simulink model "TST_EnvP_DD"  (R2016b)
settings: Solver=FixedStepDiscrete  StartTime=0.0  StopTime=simTime  FixedStep=sampleTime  RelTol=1e-3
values from neighbouring files (symbols this model uses):
  testCase = 1    [initTST_EnvP_DD_001.m]    (also in initTST_EnvP_DD_002.m = 2; initTST_EnvP_DD_003.m = 3; initTST_EnvP_DD_004.m = 4)
libraries: simulink x41, UnitTest_Lib x36
settings Model: Creator=liangyunbo  LastModifiedBy=liangyunbo
settings DebuggingCC: SignalRangeChecking=error

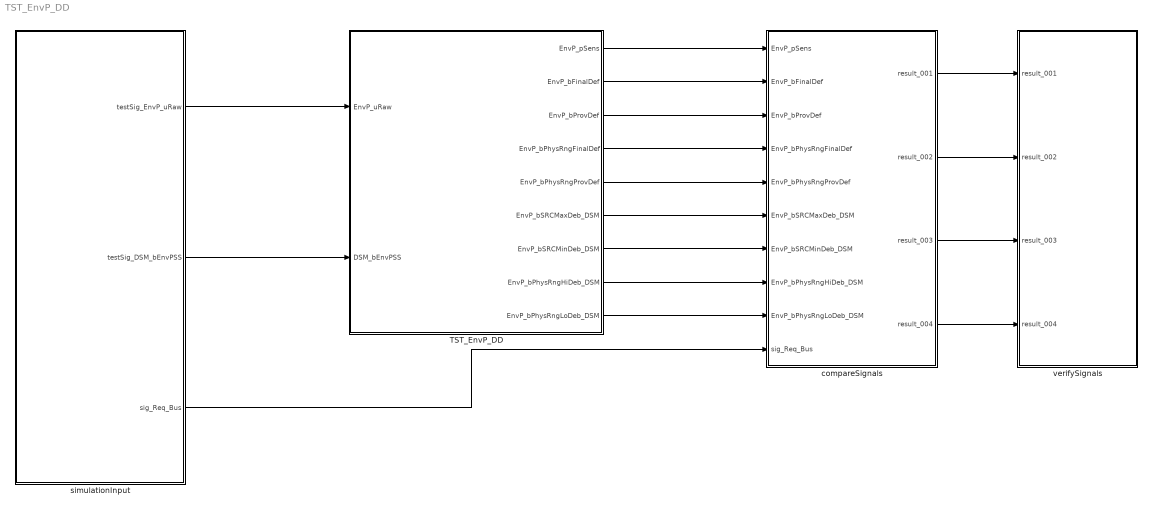
== system TST_EnvP_DD ==
  TST_EnvP_DD : Subsystem
  compareSignals : Subsystem
  simulationInput : Subsystem
  verifySignals : Subsystem
  wires:
  simulationInput/1(testSig_EnvP_uRaw) -> TST_EnvP_DD/1(EnvP_uRaw)
  simulationInput/2(testSig_DSM_bEnvPSS) -> TST_EnvP_DD/2(DSM_bEnvPSS)
  TST_EnvP_DD/1(EnvP_pSens) -> compareSignals/1(EnvP_pSens)
  TST_EnvP_DD/2(EnvP_bFinalDef) -> compareSignals/2(EnvP_bFinalDef)
  TST_EnvP_DD/3(EnvP_bProvDef) -> compareSignals/3(EnvP_bProvDef)
  TST_EnvP_DD/4(EnvP_bPhysRngFinalDef) -> compareSignals/4(EnvP_bPhysRngFinalDef)
  TST_EnvP_DD/5(EnvP_bPhysRngProvDef) -> compareSignals/5(EnvP_bPhysRngProvDef)
  TST_EnvP_DD/6(EnvP_bSRCMaxDeb_DSM) -> compareSignals/6(EnvP_bSRCMaxDeb_DSM)
  TST_EnvP_DD/7(EnvP_bSRCMinDeb_DSM) -> compareSignals/7(EnvP_bSRCMinDeb_DSM)
  TST_EnvP_DD/8(EnvP_bPhysRngHiDeb_DSM) -> compareSignals/8(EnvP_bPhysRngHiDeb_DSM)
  TST_EnvP_DD/9(EnvP_bPhysRngLoDeb_DSM) -> compareSignals/9(EnvP_bPhysRngLoDeb_DSM)
  simulationInput/3(sig_Req_Bus) -> compareSignals/10(sig_Req_Bus)
  compareSignals/1(result_001) -> verifySignals/1(result_001)
  compareSignals/2(result_002) -> verifySignals/2(result_002)
  compareSignals/3(result_003) -> verifySignals/3(result_003)
  compareSignals/4(result_004) -> verifySignals/4(result_004)

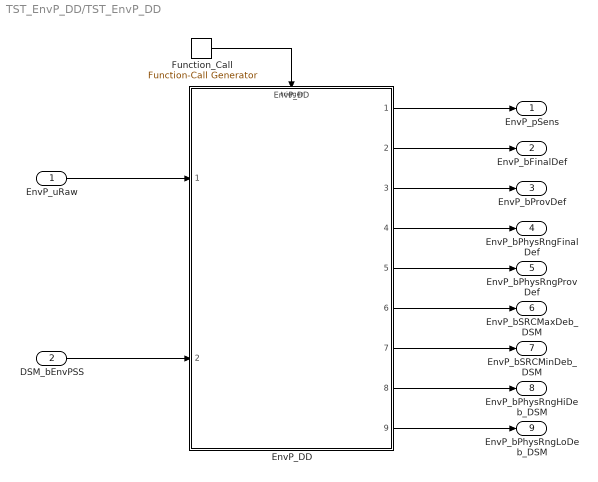
== system TST_EnvP_DD/TST_EnvP_DD ==
  EnvP_uRaw : Inport
  DSM_bEnvPSS : Inport  Port=2
  EnvP_DD : ModelReference  ModelNameDialog=EnvP_DD  SimulationMode=Normal  ModelReferenceVersion=1.9  TriggerPortName=function  TriggerPortTriggerType=function-call  TriggerPortStatesWhenEnabling=held
  Function_Call : simulink/Ports & Subsystems/Function-Call Generator  sample_time=sampleTime  numberOfIterations=1
  EnvP_pSens : Outport
  EnvP_bFinalDef : Outport  Port=2
  EnvP_bProvDef : Outport  Port=3
  EnvP_bPhysRngFinalDef : Outport  Port=4
  EnvP_bPhysRngProvDef : Outport  Port=5
  EnvP_bSRCMaxDeb_DSM : Outport  Port=6
  EnvP_bSRCMinDeb_DSM : Outport  Port=7
  EnvP_bPhysRngHiDeb_DSM : Outport  Port=8
  EnvP_bPhysRngLoDeb_DSM : Outport  Port=9
  wires:
  Function_Call/1 -> EnvP_DD/Trigger
  EnvP_uRaw/1 -> EnvP_DD/1
  DSM_bEnvPSS/1 -> EnvP_DD/2
  EnvP_DD/1 -> EnvP_pSens/1
  EnvP_DD/2 -> EnvP_bFinalDef/1
  EnvP_DD/3 -> EnvP_bProvDef/1
  EnvP_DD/4 -> EnvP_bPhysRngFinalDef/1
  EnvP_DD/5 -> EnvP_bPhysRngProvDef/1
  EnvP_DD/6 -> EnvP_bSRCMaxDeb_DSM/1
  EnvP_DD/7 -> EnvP_bSRCMinDeb_DSM/1
  EnvP_DD/8 -> EnvP_bPhysRngHiDeb_DSM/1
  EnvP_DD/9 -> EnvP_bPhysRngLoDeb_DSM/1

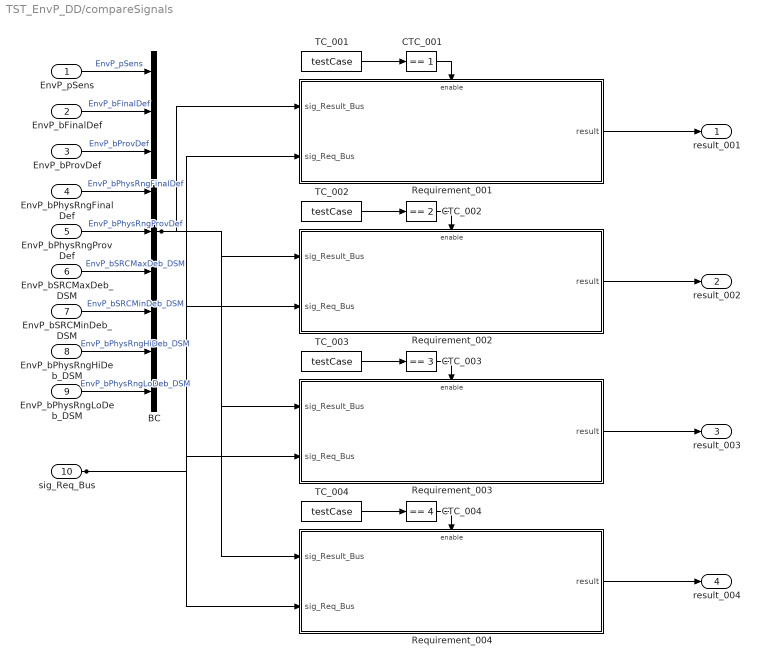
== system TST_EnvP_DD/compareSignals ==
  EnvP_pSens : Inport
  EnvP_bFinalDef : Inport  Port=2
  EnvP_bProvDef : Inport  Port=3
  EnvP_bPhysRngFinalDef : Inport  Port=4
  EnvP_bPhysRngProvDef : Inport  Port=5
  EnvP_bSRCMaxDeb_DSM : Inport  Port=6
  EnvP_bSRCMinDeb_DSM : Inport  Port=7
  EnvP_bPhysRngHiDeb_DSM : Inport  Port=8
  EnvP_bPhysRngLoDeb_DSM : Inport  Port=9
  sig_Req_Bus : Inport  Port=10
  BC : BusCreator  Inputs=9
  CTC_001 : simulink/Logic and Bit Operations/Compare To Constant  relop===  const=1  OutDataTypeStr=boolean
  CTC_002 : simulink/Logic and Bit Operations/Compare To Constant  relop===  const=2  OutDataTypeStr=boolean
  CTC_003 : simulink/Logic and Bit Operations/Compare To Constant  relop===  const=3  OutDataTypeStr=boolean
  CTC_004 : simulink/Logic and Bit Operations/Compare To Constant  relop===  const=4  OutDataTypeStr=boolean
  Requirement_001 : Subsystem
  Requirement_002 : Subsystem
  Requirement_003 : Subsystem
  Requirement_004 : Subsystem
  TC_001 : Constant  Value=testCase
  TC_002 : Constant  Value=testCase
  TC_003 : Constant  Value=testCase
  TC_004 : Constant  Value=testCase
  result_001 : Outport
  result_002 : Outport  Port=2
  result_003 : Outport  Port=3
  result_004 : Outport  Port=4
  wires:
  EnvP_pSens/1 -> BC/1  "EnvP_pSens"
  EnvP_bFinalDef/1 -> BC/2  "EnvP_bFinalDef"
  EnvP_bProvDef/1 -> BC/3  "EnvP_bProvDef"
  EnvP_bPhysRngFinalDef/1 -> BC/4  "EnvP_bPhysRngFinalDef"
  EnvP_bPhysRngProvDef/1 -> BC/5  "EnvP_bPhysRngProvDef"
  EnvP_bSRCMaxDeb_DSM/1 -> BC/6  "EnvP_bSRCMaxDeb_DSM"
  EnvP_bSRCMinDeb_DSM/1 -> BC/7  "EnvP_bSRCMinDeb_DSM"
  EnvP_bPhysRngHiDeb_DSM/1 -> BC/8  "EnvP_bPhysRngHiDeb_DSM"
  EnvP_bPhysRngLoDeb_DSM/1 -> BC/9  "EnvP_bPhysRngLoDeb_DSM"
  TC_001/1 -> CTC_001/1
  CTC_001/1 -> Requirement_001/Enable
  sig_Req_Bus/1 -> Requirement_001/2(sig_Req_Bus), Requirement_002/2(sig_Req_Bus), Requirement_003/2(sig_Req_Bus), Requirement_004/2(sig_Req_Bus)
  BC/1 -> Requirement_001/1(sig_Result_Bus), Requirement_002/1(sig_Result_Bus), Requirement_003/1(sig_Result_Bus), Requirement_004/1(sig_Result_Bus)
  Requirement_001/1(result) -> result_001/1
  TC_002/1 -> CTC_002/1
  CTC_002/1 -> Requirement_002/Enable
  Requirement_002/1(result) -> result_002/1
  TC_003/1 -> CTC_003/1
  CTC_003/1 -> Requirement_003/Enable
  Requirement_003/1(result) -> result_003/1
  TC_004/1 -> CTC_004/1
  CTC_004/1 -> Requirement_004/Enable
  Requirement_004/1(result) -> result_004/1

== system TST_EnvP_DD/simulationInput ==
  BS : BusSelector  OutputSignals=testSig_EnvP_uRaw,testSig_DSM_bEnvPSS
  MPSw : MultiPortSwitch  Inputs=4  SaturateOnIntegerOverflow=on  InputSameDT=on
  TestCase : Constant  Value=testCase
  testSignals_R001 : Subsystem
  testSignals_R002 : Subsystem
  testSignals_R003 : Subsystem
  testSignals_R004 : Subsystem
  testSig_EnvP_uRaw : Outport
  testSig_DSM_bEnvPSS : Outport  Port=2
  sig_Req_Bus : Outport  Port=3
  wires:
  BS/1 -> testSig_EnvP_uRaw/1  "<testSig_EnvP_uRaw>"
  BS/2 -> testSig_DSM_bEnvPSS/1  "<testSig_DSM_bEnvPSS>"
  MPSw/1 -> BS/1, sig_Req_Bus/1
  TestCase/1 -> MPSw/1
  testSignals_R001/1(testSignals) -> MPSw/2
  testSignals_R002/1(testSignals) -> MPSw/3
  testSignals_R003/1(testSignals) -> MPSw/4
  testSignals_R004/1(testSignals) -> MPSw/5

== system TST_EnvP_DD/verifySignals ==
  result_001 : Inport
  result_002 : Inport  Port=2
  result_003 : Inport  Port=3
  result_004 : Inport  Port=4
  Assertion_001 : Assertion  Enabled=off
  Assertion_002 : Assertion  Enabled=off
  Assertion_003 : Assertion  Enabled=off
  Assertion_004 : Assertion  Enabled=off
  wires:
  result_001/1 -> Assertion_001/1
  result_002/1 -> Assertion_002/1
  result_003/1 -> Assertion_003/1
  result_004/1 -> Assertion_004/1

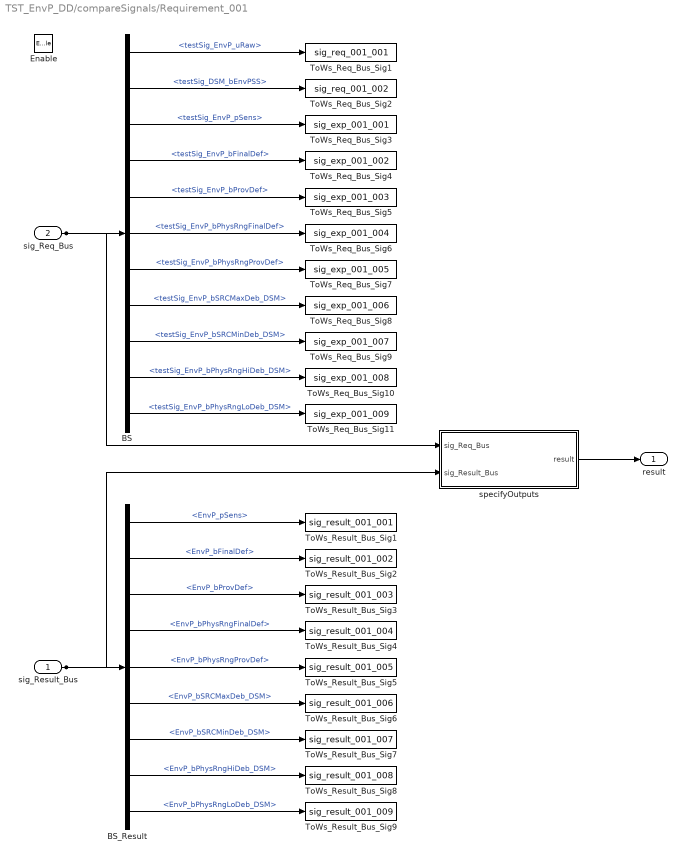
== system TST_EnvP_DD/compareSignals/Requirement_001 ==
  sig_Result_Bus : Inport
  sig_Req_Bus : Inport  Port=2
  Enable : EnablePort
  BS : BusSelector  OutputSignals=testSig_EnvP_uRaw,testSig_DSM_bEnvPSS,testSig_EnvP_pSens,testSig_EnvP_bFinalDef,testSig_EnvP_bProvDef,testSig_EnvP_bPhysRngFinalDef,testSig_EnvP_bPhysRngProvDef,testSig_EnvP_bSRCMaxDeb_DSM,testSig_EnvP_bSRCMinDeb_DSM,testSig_EnvP_bPhysRngHiDeb_DSM,testSig_EnvP_bPhysRngLoDeb_DSM
  BS_Result : BusSelector  OutputSignals=EnvP_pSens,EnvP_bFinalDef,EnvP_bProvDef,EnvP_bPhysRngFinalDef,EnvP_bPhysRngProvDef,EnvP_bSRCMaxDeb_DSM,EnvP_bSRCMinDeb_DSM,EnvP_bPhysRngHiDeb_DSM,EnvP_bPhysRngLoDeb_DSM
  ToWs_Req_Bus_Sig1 : ToWorkspace  VariableName=sig_req_001_001  SaveFormat=Structure With Time
  ToWs_Req_Bus_Sig10 : ToWorkspace  VariableName=sig_exp_001_008  SaveFormat=Structure With Time
  ToWs_Req_Bus_Sig11 : ToWorkspace  VariableName=sig_exp_001_009  SaveFormat=Structure With Time
  ToWs_Req_Bus_Sig2 : ToWorkspace  VariableName=sig_req_001_002  SaveFormat=Structure With Time
  ToWs_Req_Bus_Sig3 : ToWorkspace  VariableName=sig_exp_001_001  SaveFormat=Structure With Time
  ToWs_Req_Bus_Sig4 : ToWorkspace  VariableName=sig_exp_001_002  SaveFormat=Structure With Time
  ToWs_Req_Bus_Sig5 : ToWorkspace  VariableName=sig_exp_001_003  SaveFormat=Structure With Time
  ToWs_Req_Bus_Sig6 : ToWorkspace  VariableName=sig_exp_001_004  SaveFormat=Structure With Time
  ToWs_Req_Bus_Sig7 : ToWorkspace  VariableName=sig_exp_001_005  SaveFormat=Structure With Time
  ToWs_Req_Bus_Sig8 : ToWorkspace  VariableName=sig_exp_001_006  SaveFormat=Structure With Time
  ToWs_Req_Bus_Sig9 : ToWorkspace  VariableName=sig_exp_001_007  SaveFormat=Structure With Time
  ToWs_Result_Bus_Sig1 : ToWorkspace  VariableName=sig_result_001_001  SaveFormat=Structure With Time
  ToWs_Result_Bus_Sig2 : ToWorkspace  VariableName=sig_result_001_002  SaveFormat=Structure With Time
  ToWs_Result_Bus_Sig3 : ToWorkspace  VariableName=sig_result_001_003  SaveFormat=Structure With Time
  ToWs_Result_Bus_Sig4 : ToWorkspace  VariableName=sig_result_001_004  SaveFormat=Structure With Time
  ToWs_Result_Bus_Sig5 : ToWorkspace  VariableName=sig_result_001_005  SaveFormat=Structure With Time
  ToWs_Result_Bus_Sig6 : ToWorkspace  VariableName=sig_result_001_006  SaveFormat=Structure With Time
  ToWs_Result_Bus_Sig7 : ToWorkspace  VariableName=sig_result_001_007  SaveFormat=Structure With Time
  ToWs_Result_Bus_Sig8 : ToWorkspace  VariableName=sig_result_001_008  SaveFormat=Structure With Time
  ToWs_Result_Bus_Sig9 : ToWorkspace  VariableName=sig_result_001_009  SaveFormat=Structure With Time
  specifyOutputs : Subsystem
  result : Outport
  wires:
  sig_Req_Bus/1 -> BS/1, specifyOutputs/1(sig_Req_Bus)
  BS/1 -> ToWs_Req_Bus_Sig1/1  "<testSig_EnvP_uRaw>"
  BS/2 -> ToWs_Req_Bus_Sig2/1  "<testSig_DSM_bEnvPSS>"
  BS/3 -> ToWs_Req_Bus_Sig3/1  "<testSig_EnvP_pSens>"
  BS/4 -> ToWs_Req_Bus_Sig4/1  "<testSig_EnvP_bFinalDef>"
  BS/5 -> ToWs_Req_Bus_Sig5/1  "<testSig_EnvP_bProvDef>"
  BS/6 -> ToWs_Req_Bus_Sig6/1  "<testSig_EnvP_bPhysRngFinalDef>"
  BS/7 -> ToWs_Req_Bus_Sig7/1  "<testSig_EnvP_bPhysRngProvDef>"
  BS/8 -> ToWs_Req_Bus_Sig8/1  "<testSig_EnvP_bSRCMaxDeb_DSM>"
  BS/9 -> ToWs_Req_Bus_Sig9/1  "<testSig_EnvP_bSRCMinDeb_DSM>"
  BS/10 -> ToWs_Req_Bus_Sig10/1  "<testSig_EnvP_bPhysRngHiDeb_DSM>"
  BS/11 -> ToWs_Req_Bus_Sig11/1  "<testSig_EnvP_bPhysRngLoDeb_DSM>"
  sig_Result_Bus/1 -> BS_Result/1, specifyOutputs/2(sig_Result_Bus)
  BS_Result/1 -> ToWs_Result_Bus_Sig1/1  "<EnvP_pSens>"
  BS_Result/2 -> ToWs_Result_Bus_Sig2/1  "<EnvP_bFinalDef>"
  BS_Result/3 -> ToWs_Result_Bus_Sig3/1  "<EnvP_bProvDef>"
  BS_Result/4 -> ToWs_Result_Bus_Sig4/1  "<EnvP_bPhysRngFinalDef>"
  BS_Result/5 -> ToWs_Result_Bus_Sig5/1  "<EnvP_bPhysRngProvDef>"
  BS_Result/6 -> ToWs_Result_Bus_Sig6/1  "<EnvP_bSRCMaxDeb_DSM>"
  BS_Result/7 -> ToWs_Result_Bus_Sig7/1  "<EnvP_bSRCMinDeb_DSM>"
  BS_Result/8 -> ToWs_Result_Bus_Sig8/1  "<EnvP_bPhysRngHiDeb_DSM>"
  BS_Result/9 -> ToWs_Result_Bus_Sig9/1  "<EnvP_bPhysRngLoDeb_DSM>"
  specifyOutputs/1(result) -> result/1

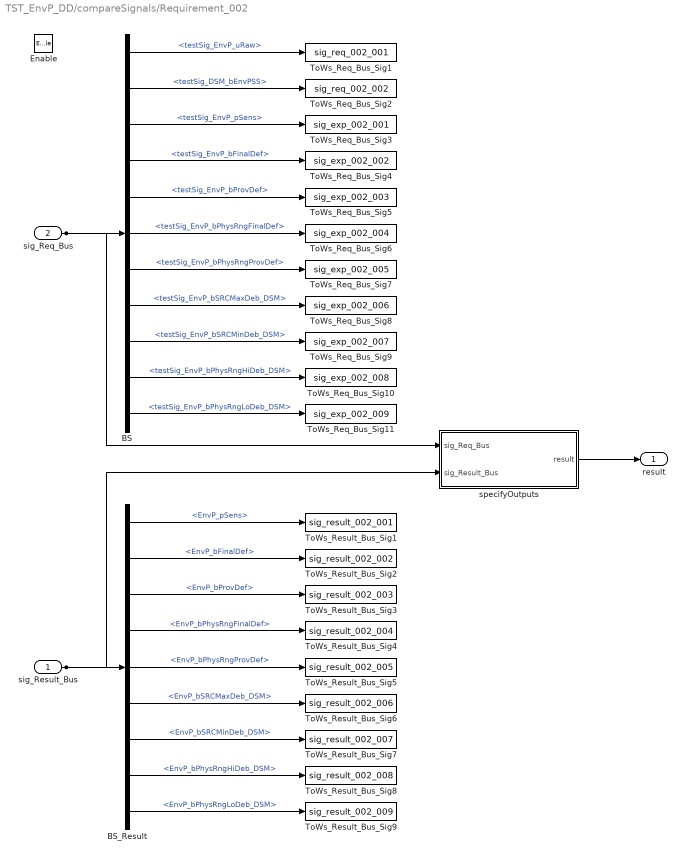
== system TST_EnvP_DD/compareSignals/Requirement_002 ==
  sig_Result_Bus : Inport
  sig_Req_Bus : Inport  Port=2
  Enable : EnablePort
  BS : BusSelector  OutputSignals=testSig_EnvP_uRaw,testSig_DSM_bEnvPSS,testSig_EnvP_pSens,testSig_EnvP_bFinalDef,testSig_EnvP_bProvDef,testSig_EnvP_bPhysRngFinalDef,testSig_EnvP_bPhysRngProvDef,testSig_EnvP_bSRCMaxDeb_DSM,testSig_EnvP_bSRCMinDeb_DSM,testSig_EnvP_bPhysRngHiDeb_DSM,testSig_EnvP_bPhysRngLoDeb_DSM
  BS_Result : BusSelector  OutputSignals=EnvP_pSens,EnvP_bFinalDef,EnvP_bProvDef,EnvP_bPhysRngFinalDef,EnvP_bPhysRngProvDef,EnvP_bSRCMaxDeb_DSM,EnvP_bSRCMinDeb_DSM,EnvP_bPhysRngHiDeb_DSM,EnvP_bPhysRngLoDeb_DSM
  ToWs_Req_Bus_Sig1 : ToWorkspace  VariableName=sig_req_002_001  SaveFormat=Structure With Time
  ToWs_Req_Bus_Sig10 : ToWorkspace  VariableName=sig_exp_002_008  SaveFormat=Structure With Time
  ToWs_Req_Bus_Sig11 : ToWorkspace  VariableName=sig_exp_002_009  SaveFormat=Structure With Time
  ToWs_Req_Bus_Sig2 : ToWorkspace  VariableName=sig_req_002_002  SaveFormat=Structure With Time
  ToWs_Req_Bus_Sig3 : ToWorkspace  VariableName=sig_exp_002_001  SaveFormat=Structure With Time
  ToWs_Req_Bus_Sig4 : ToWorkspace  VariableName=sig_exp_002_002  SaveFormat=Structure With Time
  ToWs_Req_Bus_Sig5 : ToWorkspace  VariableName=sig_exp_002_003  SaveFormat=Structure With Time
  ToWs_Req_Bus_Sig6 : ToWorkspace  VariableName=sig_exp_002_004  SaveFormat=Structure With Time
  ToWs_Req_Bus_Sig7 : ToWorkspace  VariableName=sig_exp_002_005  SaveFormat=Structure With Time
  ToWs_Req_Bus_Sig8 : ToWorkspace  VariableName=sig_exp_002_006  SaveFormat=Structure With Time
  ToWs_Req_Bus_Sig9 : ToWorkspace  VariableName=sig_exp_002_007  SaveFormat=Structure With Time
  ToWs_Result_Bus_Sig1 : ToWorkspace  VariableName=sig_result_002_001  SaveFormat=Structure With Time
  ToWs_Result_Bus_Sig2 : ToWorkspace  VariableName=sig_result_002_002  SaveFormat=Structure With Time
  ToWs_Result_Bus_Sig3 : ToWorkspace  VariableName=sig_result_002_003  SaveFormat=Structure With Time
  ToWs_Result_Bus_Sig4 : ToWorkspace  VariableName=sig_result_002_004  SaveFormat=Structure With Time
  ToWs_Result_Bus_Sig5 : ToWorkspace  VariableName=sig_result_002_005  SaveFormat=Structure With Time
  ToWs_Result_Bus_Sig6 : ToWorkspace  VariableName=sig_result_002_006  SaveFormat=Structure With Time
  ToWs_Result_Bus_Sig7 : ToWorkspace  VariableName=sig_result_002_007  SaveFormat=Structure With Time
  ToWs_Result_Bus_Sig8 : ToWorkspace  VariableName=sig_result_002_008  SaveFormat=Structure With Time
  ToWs_Result_Bus_Sig9 : ToWorkspace  VariableName=sig_result_002_009  SaveFormat=Structure With Time
  specifyOutputs : Subsystem
  result : Outport
  wires:
  sig_Req_Bus/1 -> BS/1, specifyOutputs/1(sig_Req_Bus)
  BS/1 -> ToWs_Req_Bus_Sig1/1  "<testSig_EnvP_uRaw>"
  BS/2 -> ToWs_Req_Bus_Sig2/1  "<testSig_DSM_bEnvPSS>"
  BS/3 -> ToWs_Req_Bus_Sig3/1  "<testSig_EnvP_pSens>"
  BS/4 -> ToWs_Req_Bus_Sig4/1  "<testSig_EnvP_bFinalDef>"
  BS/5 -> ToWs_Req_Bus_Sig5/1  "<testSig_EnvP_bProvDef>"
  BS/6 -> ToWs_Req_Bus_Sig6/1  "<testSig_EnvP_bPhysRngFinalDef>"
  BS/7 -> ToWs_Req_Bus_Sig7/1  "<testSig_EnvP_bPhysRngProvDef>"
  BS/8 -> ToWs_Req_Bus_Sig8/1  "<testSig_EnvP_bSRCMaxDeb_DSM>"
  BS/9 -> ToWs_Req_Bus_Sig9/1  "<testSig_EnvP_bSRCMinDeb_DSM>"
  BS/10 -> ToWs_Req_Bus_Sig10/1  "<testSig_EnvP_bPhysRngHiDeb_DSM>"
  BS/11 -> ToWs_Req_Bus_Sig11/1  "<testSig_EnvP_bPhysRngLoDeb_DSM>"
  sig_Result_Bus/1 -> BS_Result/1, specifyOutputs/2(sig_Result_Bus)
  BS_Result/1 -> ToWs_Result_Bus_Sig1/1  "<EnvP_pSens>"
  BS_Result/2 -> ToWs_Result_Bus_Sig2/1  "<EnvP_bFinalDef>"
  BS_Result/3 -> ToWs_Result_Bus_Sig3/1  "<EnvP_bProvDef>"
  BS_Result/4 -> ToWs_Result_Bus_Sig4/1  "<EnvP_bPhysRngFinalDef>"
  BS_Result/5 -> ToWs_Result_Bus_Sig5/1  "<EnvP_bPhysRngProvDef>"
  BS_Result/6 -> ToWs_Result_Bus_Sig6/1  "<EnvP_bSRCMaxDeb_DSM>"
  BS_Result/7 -> ToWs_Result_Bus_Sig7/1  "<EnvP_bSRCMinDeb_DSM>"
  BS_Result/8 -> ToWs_Result_Bus_Sig8/1  "<EnvP_bPhysRngHiDeb_DSM>"
  BS_Result/9 -> ToWs_Result_Bus_Sig9/1  "<EnvP_bPhysRngLoDeb_DSM>"
  specifyOutputs/1(result) -> result/1

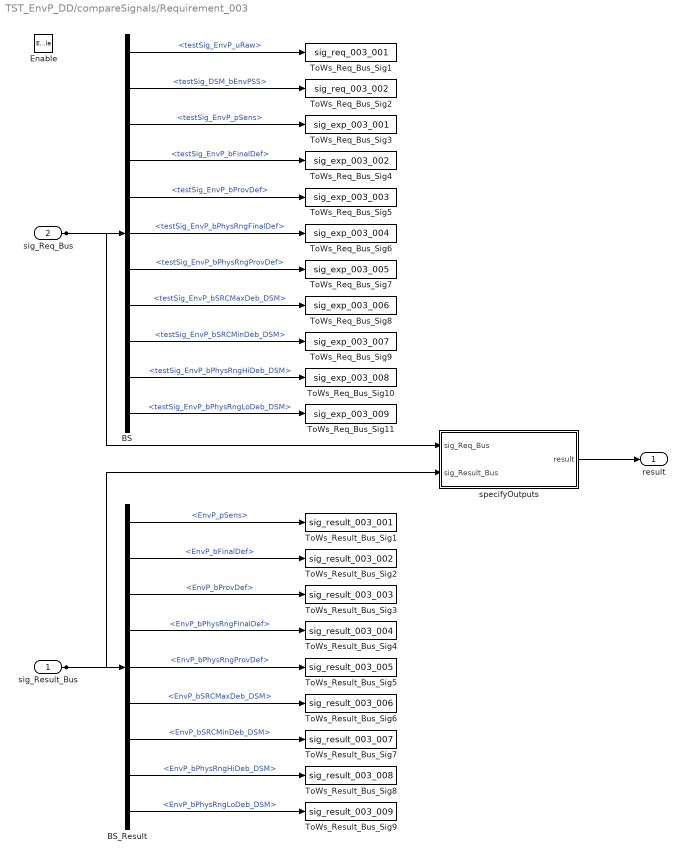
== system TST_EnvP_DD/compareSignals/Requirement_003 ==
  sig_Result_Bus : Inport
  sig_Req_Bus : Inport  Port=2
  Enable : EnablePort
  BS : BusSelector  OutputSignals=testSig_EnvP_uRaw,testSig_DSM_bEnvPSS,testSig_EnvP_pSens,testSig_EnvP_bFinalDef,testSig_EnvP_bProvDef,testSig_EnvP_bPhysRngFinalDef,testSig_EnvP_bPhysRngProvDef,testSig_EnvP_bSRCMaxDeb_DSM,testSig_EnvP_bSRCMinDeb_DSM,testSig_EnvP_bPhysRngHiDeb_DSM,testSig_EnvP_bPhysRngLoDeb_DSM
  BS_Result : BusSelector  OutputSignals=EnvP_pSens,EnvP_bFinalDef,EnvP_bProvDef,EnvP_bPhysRngFinalDef,EnvP_bPhysRngProvDef,EnvP_bSRCMaxDeb_DSM,EnvP_bSRCMinDeb_DSM,EnvP_bPhysRngHiDeb_DSM,EnvP_bPhysRngLoDeb_DSM
  ToWs_Req_Bus_Sig1 : ToWorkspace  VariableName=sig_req_003_001  SaveFormat=Structure With Time
  ToWs_Req_Bus_Sig10 : ToWorkspace  VariableName=sig_exp_003_008  SaveFormat=Structure With Time
  ToWs_Req_Bus_Sig11 : ToWorkspace  VariableName=sig_exp_003_009  SaveFormat=Structure With Time
  ToWs_Req_Bus_Sig2 : ToWorkspace  VariableName=sig_req_003_002  SaveFormat=Structure With Time
  ToWs_Req_Bus_Sig3 : ToWorkspace  VariableName=sig_exp_003_001  SaveFormat=Structure With Time
  ToWs_Req_Bus_Sig4 : ToWorkspace  VariableName=sig_exp_003_002  SaveFormat=Structure With Time
  ToWs_Req_Bus_Sig5 : ToWorkspace  VariableName=sig_exp_003_003  SaveFormat=Structure With Time
  ToWs_Req_Bus_Sig6 : ToWorkspace  VariableName=sig_exp_003_004  SaveFormat=Structure With Time
  ToWs_Req_Bus_Sig7 : ToWorkspace  VariableName=sig_exp_003_005  SaveFormat=Structure With Time
  ToWs_Req_Bus_Sig8 : ToWorkspace  VariableName=sig_exp_003_006  SaveFormat=Structure With Time
  ToWs_Req_Bus_Sig9 : ToWorkspace  VariableName=sig_exp_003_007  SaveFormat=Structure With Time
  ToWs_Result_Bus_Sig1 : ToWorkspace  VariableName=sig_result_003_001  SaveFormat=Structure With Time
  ToWs_Result_Bus_Sig2 : ToWorkspace  VariableName=sig_result_003_002  SaveFormat=Structure With Time
  ToWs_Result_Bus_Sig3 : ToWorkspace  VariableName=sig_result_003_003  SaveFormat=Structure With Time
  ToWs_Result_Bus_Sig4 : ToWorkspace  VariableName=sig_result_003_004  SaveFormat=Structure With Time
  ToWs_Result_Bus_Sig5 : ToWorkspace  VariableName=sig_result_003_005  SaveFormat=Structure With Time
  ToWs_Result_Bus_Sig6 : ToWorkspace  VariableName=sig_result_003_006  SaveFormat=Structure With Time
  ToWs_Result_Bus_Sig7 : ToWorkspace  VariableName=sig_result_003_007  SaveFormat=Structure With Time
  ToWs_Result_Bus_Sig8 : ToWorkspace  VariableName=sig_result_003_008  SaveFormat=Structure With Time
  ToWs_Result_Bus_Sig9 : ToWorkspace  VariableName=sig_result_003_009  SaveFormat=Structure With Time
  specifyOutputs : Subsystem
  result : Outport
  wires:
  sig_Req_Bus/1 -> BS/1, specifyOutputs/1(sig_Req_Bus)
  BS/1 -> ToWs_Req_Bus_Sig1/1  "<testSig_EnvP_uRaw>"
  BS/2 -> ToWs_Req_Bus_Sig2/1  "<testSig_DSM_bEnvPSS>"
  BS/3 -> ToWs_Req_Bus_Sig3/1  "<testSig_EnvP_pSens>"
  BS/4 -> ToWs_Req_Bus_Sig4/1  "<testSig_EnvP_bFinalDef>"
  BS/5 -> ToWs_Req_Bus_Sig5/1  "<testSig_EnvP_bProvDef>"
  BS/6 -> ToWs_Req_Bus_Sig6/1  "<testSig_EnvP_bPhysRngFinalDef>"
  BS/7 -> ToWs_Req_Bus_Sig7/1  "<testSig_EnvP_bPhysRngProvDef>"
  BS/8 -> ToWs_Req_Bus_Sig8/1  "<testSig_EnvP_bSRCMaxDeb_DSM>"
  BS/9 -> ToWs_Req_Bus_Sig9/1  "<testSig_EnvP_bSRCMinDeb_DSM>"
  BS/10 -> ToWs_Req_Bus_Sig10/1  "<testSig_EnvP_bPhysRngHiDeb_DSM>"
  BS/11 -> ToWs_Req_Bus_Sig11/1  "<testSig_EnvP_bPhysRngLoDeb_DSM>"
  sig_Result_Bus/1 -> BS_Result/1, specifyOutputs/2(sig_Result_Bus)
  BS_Result/1 -> ToWs_Result_Bus_Sig1/1  "<EnvP_pSens>"
  BS_Result/2 -> ToWs_Result_Bus_Sig2/1  "<EnvP_bFinalDef>"
  BS_Result/3 -> ToWs_Result_Bus_Sig3/1  "<EnvP_bProvDef>"
  BS_Result/4 -> ToWs_Result_Bus_Sig4/1  "<EnvP_bPhysRngFinalDef>"
  BS_Result/5 -> ToWs_Result_Bus_Sig5/1  "<EnvP_bPhysRngProvDef>"
  BS_Result/6 -> ToWs_Result_Bus_Sig6/1  "<EnvP_bSRCMaxDeb_DSM>"
  BS_Result/7 -> ToWs_Result_Bus_Sig7/1  "<EnvP_bSRCMinDeb_DSM>"
  BS_Result/8 -> ToWs_Result_Bus_Sig8/1  "<EnvP_bPhysRngHiDeb_DSM>"
  BS_Result/9 -> ToWs_Result_Bus_Sig9/1  "<EnvP_bPhysRngLoDeb_DSM>"
  specifyOutputs/1(result) -> result/1

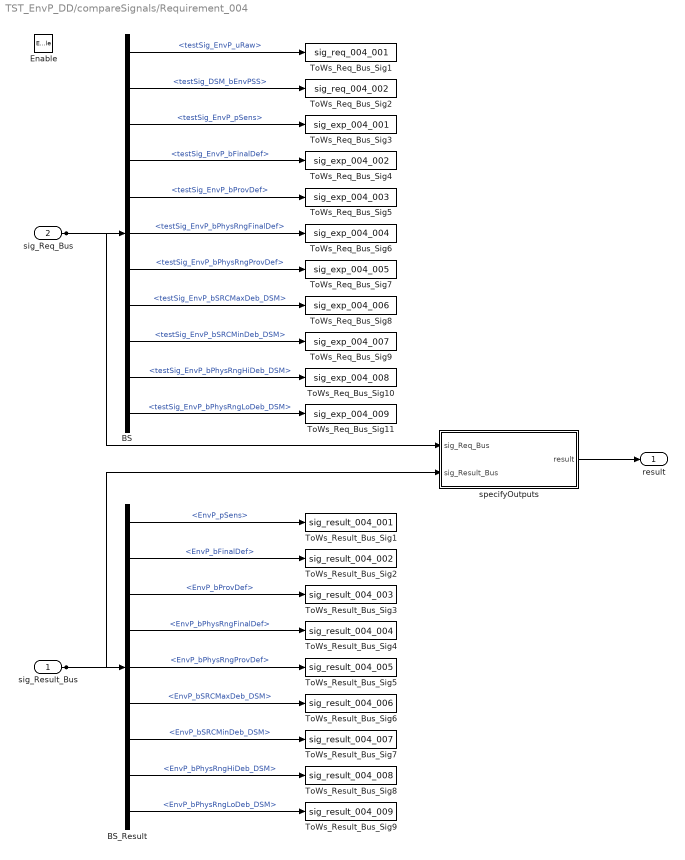
== system TST_EnvP_DD/compareSignals/Requirement_004 ==
  sig_Result_Bus : Inport
  sig_Req_Bus : Inport  Port=2
  Enable : EnablePort
  BS : BusSelector  OutputSignals=testSig_EnvP_uRaw,testSig_DSM_bEnvPSS,testSig_EnvP_pSens,testSig_EnvP_bFinalDef,testSig_EnvP_bProvDef,testSig_EnvP_bPhysRngFinalDef,testSig_EnvP_bPhysRngProvDef,testSig_EnvP_bSRCMaxDeb_DSM,testSig_EnvP_bSRCMinDeb_DSM,testSig_EnvP_bPhysRngHiDeb_DSM,testSig_EnvP_bPhysRngLoDeb_DSM
  BS_Result : BusSelector  OutputSignals=EnvP_pSens,EnvP_bFinalDef,EnvP_bProvDef,EnvP_bPhysRngFinalDef,EnvP_bPhysRngProvDef,EnvP_bSRCMaxDeb_DSM,EnvP_bSRCMinDeb_DSM,EnvP_bPhysRngHiDeb_DSM,EnvP_bPhysRngLoDeb_DSM
  ToWs_Req_Bus_Sig1 : ToWorkspace  VariableName=sig_req_004_001  SaveFormat=Structure With Time
  ToWs_Req_Bus_Sig10 : ToWorkspace  VariableName=sig_exp_004_008  SaveFormat=Structure With Time
  ToWs_Req_Bus_Sig11 : ToWorkspace  VariableName=sig_exp_004_009  SaveFormat=Structure With Time
  ToWs_Req_Bus_Sig2 : ToWorkspace  VariableName=sig_req_004_002  SaveFormat=Structure With Time
  ToWs_Req_Bus_Sig3 : ToWorkspace  VariableName=sig_exp_004_001  SaveFormat=Structure With Time
  ToWs_Req_Bus_Sig4 : ToWorkspace  VariableName=sig_exp_004_002  SaveFormat=Structure With Time
  ToWs_Req_Bus_Sig5 : ToWorkspace  VariableName=sig_exp_004_003  SaveFormat=Structure With Time
  ToWs_Req_Bus_Sig6 : ToWorkspace  VariableName=sig_exp_004_004  SaveFormat=Structure With Time
  ToWs_Req_Bus_Sig7 : ToWorkspace  VariableName=sig_exp_004_005  SaveFormat=Structure With Time
  ToWs_Req_Bus_Sig8 : ToWorkspace  VariableName=sig_exp_004_006  SaveFormat=Structure With Time
  ToWs_Req_Bus_Sig9 : ToWorkspace  VariableName=sig_exp_004_007  SaveFormat=Structure With Time
  ToWs_Result_Bus_Sig1 : ToWorkspace  VariableName=sig_result_004_001  SaveFormat=Structure With Time
  ToWs_Result_Bus_Sig2 : ToWorkspace  VariableName=sig_result_004_002  SaveFormat=Structure With Time
  ToWs_Result_Bus_Sig3 : ToWorkspace  VariableName=sig_result_004_003  SaveFormat=Structure With Time
  ToWs_Result_Bus_Sig4 : ToWorkspace  VariableName=sig_result_004_004  SaveFormat=Structure With Time
  ToWs_Result_Bus_Sig5 : ToWorkspace  VariableName=sig_result_004_005  SaveFormat=Structure With Time
  ToWs_Result_Bus_Sig6 : ToWorkspace  VariableName=sig_result_004_006  SaveFormat=Structure With Time
  ToWs_Result_Bus_Sig7 : ToWorkspace  VariableName=sig_result_004_007  SaveFormat=Structure With Time
  ToWs_Result_Bus_Sig8 : ToWorkspace  VariableName=sig_result_004_008  SaveFormat=Structure With Time
  ToWs_Result_Bus_Sig9 : ToWorkspace  VariableName=sig_result_004_009  SaveFormat=Structure With Time
  specifyOutputs : Subsystem
  result : Outport
  wires:
  sig_Req_Bus/1 -> BS/1, specifyOutputs/1(sig_Req_Bus)
  BS/1 -> ToWs_Req_Bus_Sig1/1  "<testSig_EnvP_uRaw>"
  BS/2 -> ToWs_Req_Bus_Sig2/1  "<testSig_DSM_bEnvPSS>"
  BS/3 -> ToWs_Req_Bus_Sig3/1  "<testSig_EnvP_pSens>"
  BS/4 -> ToWs_Req_Bus_Sig4/1  "<testSig_EnvP_bFinalDef>"
  BS/5 -> ToWs_Req_Bus_Sig5/1  "<testSig_EnvP_bProvDef>"
  BS/6 -> ToWs_Req_Bus_Sig6/1  "<testSig_EnvP_bPhysRngFinalDef>"
  BS/7 -> ToWs_Req_Bus_Sig7/1  "<testSig_EnvP_bPhysRngProvDef>"
  BS/8 -> ToWs_Req_Bus_Sig8/1  "<testSig_EnvP_bSRCMaxDeb_DSM>"
  BS/9 -> ToWs_Req_Bus_Sig9/1  "<testSig_EnvP_bSRCMinDeb_DSM>"
  BS/10 -> ToWs_Req_Bus_Sig10/1  "<testSig_EnvP_bPhysRngHiDeb_DSM>"
  BS/11 -> ToWs_Req_Bus_Sig11/1  "<testSig_EnvP_bPhysRngLoDeb_DSM>"
  sig_Result_Bus/1 -> BS_Result/1, specifyOutputs/2(sig_Result_Bus)
  BS_Result/1 -> ToWs_Result_Bus_Sig1/1  "<EnvP_pSens>"
  BS_Result/2 -> ToWs_Result_Bus_Sig2/1  "<EnvP_bFinalDef>"
  BS_Result/3 -> ToWs_Result_Bus_Sig3/1  "<EnvP_bProvDef>"
  BS_Result/4 -> ToWs_Result_Bus_Sig4/1  "<EnvP_bPhysRngFinalDef>"
  BS_Result/5 -> ToWs_Result_Bus_Sig5/1  "<EnvP_bPhysRngProvDef>"
  BS_Result/6 -> ToWs_Result_Bus_Sig6/1  "<EnvP_bSRCMaxDeb_DSM>"
  BS_Result/7 -> ToWs_Result_Bus_Sig7/1  "<EnvP_bSRCMinDeb_DSM>"
  BS_Result/8 -> ToWs_Result_Bus_Sig8/1  "<EnvP_bPhysRngHiDeb_DSM>"
  BS_Result/9 -> ToWs_Result_Bus_Sig9/1  "<EnvP_bPhysRngLoDeb_DSM>"
  specifyOutputs/1(result) -> result/1

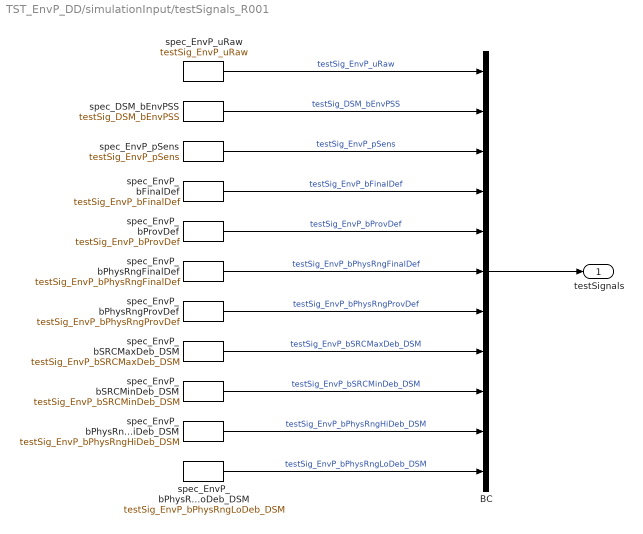
== system TST_EnvP_DD/simulationInput/testSignals_R001 ==
  BC : BusCreator  Inputs=11
  spec_DSM_bEnvPSS : FromWorkspace  VariableName=testSig_DSM_bEnvPSS  Interpolate=off  OutputAfterFinalValue=Holding final value
  spec_EnvP_bFinalDef : FromWorkspace  VariableName=testSig_EnvP_bFinalDef  Interpolate=off  OutputAfterFinalValue=Holding final value
  spec_EnvP_bPhysRngFinalDef : FromWorkspace  VariableName=testSig_EnvP_bPhysRngFinalDef  Interpolate=off  OutputAfterFinalValue=Holding final value
  spec_EnvP_bPhysRngHiDeb_DSM : FromWorkspace  VariableName=testSig_EnvP_bPhysRngHiDeb_DSM  Interpolate=off  OutputAfterFinalValue=Holding final value
  spec_EnvP_bPhysRngLoDeb_DSM : FromWorkspace  VariableName=testSig_EnvP_bPhysRngLoDeb_DSM  Interpolate=off  OutputAfterFinalValue=Holding final value
  spec_EnvP_bPhysRngProvDef : FromWorkspace  VariableName=testSig_EnvP_bPhysRngProvDef  Interpolate=off  OutputAfterFinalValue=Holding final value
  spec_EnvP_bProvDef : FromWorkspace  VariableName=testSig_EnvP_bProvDef  Interpolate=off  OutputAfterFinalValue=Holding final value
  spec_EnvP_bSRCMaxDeb_DSM : FromWorkspace  VariableName=testSig_EnvP_bSRCMaxDeb_DSM  Interpolate=off  OutputAfterFinalValue=Holding final value
  spec_EnvP_bSRCMinDeb_DSM : FromWorkspace  VariableName=testSig_EnvP_bSRCMinDeb_DSM  Interpolate=off  OutputAfterFinalValue=Holding final value
  spec_EnvP_pSens : FromWorkspace  VariableName=testSig_EnvP_pSens  Interpolate=off  OutputAfterFinalValue=Holding final value
  spec_EnvP_uRaw : FromWorkspace  VariableName=testSig_EnvP_uRaw  Interpolate=off  OutputAfterFinalValue=Holding final value
  testSignals : Outport
  wires:
  BC/1 -> testSignals/1
  spec_EnvP_uRaw/1 -> BC/1  "testSig_EnvP_uRaw"
  spec_DSM_bEnvPSS/1 -> BC/2  "testSig_DSM_bEnvPSS"
  spec_EnvP_pSens/1 -> BC/3  "testSig_EnvP_pSens"
  spec_EnvP_bFinalDef/1 -> BC/4  "testSig_EnvP_bFinalDef"
  spec_EnvP_bProvDef/1 -> BC/5  "testSig_EnvP_bProvDef"
  spec_EnvP_bPhysRngFinalDef/1 -> BC/6  "testSig_EnvP_bPhysRngFinalDef"
  spec_EnvP_bPhysRngProvDef/1 -> BC/7  "testSig_EnvP_bPhysRngProvDef"
  spec_EnvP_bSRCMaxDeb_DSM/1 -> BC/8  "testSig_EnvP_bSRCMaxDeb_DSM"
  spec_EnvP_bSRCMinDeb_DSM/1 -> BC/9  "testSig_EnvP_bSRCMinDeb_DSM"
  spec_EnvP_bPhysRngHiDeb_DSM/1 -> BC/10  "testSig_EnvP_bPhysRngHiDeb_DSM"
  spec_EnvP_bPhysRngLoDeb_DSM/1 -> BC/11  "testSig_EnvP_bPhysRngLoDeb_DSM"

== system TST_EnvP_DD/simulationInput/testSignals_R002 ==
  BC : BusCreator  Inputs=11
  spec_DSM_bEnvPSS : FromWorkspace  VariableName=testSig_DSM_bEnvPSS  Interpolate=off  OutputAfterFinalValue=Holding final value
  spec_EnvP_bFinalDef : FromWorkspace  VariableName=testSig_EnvP_bFinalDef  Interpolate=off  OutputAfterFinalValue=Holding final value
  spec_EnvP_bPhysRngFinalDef : FromWorkspace  VariableName=testSig_EnvP_bPhysRngFinalDef  Interpolate=off  OutputAfterFinalValue=Holding final value
  spec_EnvP_bPhysRngHiDeb_DSM : FromWorkspace  VariableName=testSig_EnvP_bPhysRngHiDeb_DSM  Interpolate=off  OutputAfterFinalValue=Holding final value
  spec_EnvP_bPhysRngLoDeb_DSM : FromWorkspace  VariableName=testSig_EnvP_bPhysRngLoDeb_DSM  Interpolate=off  OutputAfterFinalValue=Holding final value
  spec_EnvP_bPhysRngProvDef : FromWorkspace  VariableName=testSig_EnvP_bPhysRngProvDef  Interpolate=off  OutputAfterFinalValue=Holding final value
  spec_EnvP_bProvDef : FromWorkspace  VariableName=testSig_EnvP_bProvDef  Interpolate=off  OutputAfterFinalValue=Holding final value
  spec_EnvP_bSRCMaxDeb_DSM : FromWorkspace  VariableName=testSig_EnvP_bSRCMaxDeb_DSM  Interpolate=off  OutputAfterFinalValue=Holding final value
  spec_EnvP_bSRCMinDeb_DSM : FromWorkspace  VariableName=testSig_EnvP_bSRCMinDeb_DSM  Interpolate=off  OutputAfterFinalValue=Holding final value
  spec_EnvP_pSens : FromWorkspace  VariableName=testSig_EnvP_pSens  Interpolate=off  OutputAfterFinalValue=Holding final value
  spec_EnvP_uRaw : FromWorkspace  VariableName=testSig_EnvP_uRaw  Interpolate=off  OutputAfterFinalValue=Holding final value
  testSignals : Outport
  wires:
  BC/1 -> testSignals/1
  spec_EnvP_uRaw/1 -> BC/1  "testSig_EnvP_uRaw"
  spec_DSM_bEnvPSS/1 -> BC/2  "testSig_DSM_bEnvPSS"
  spec_EnvP_pSens/1 -> BC/3  "testSig_EnvP_pSens"
  spec_EnvP_bFinalDef/1 -> BC/4  "testSig_EnvP_bFinalDef"
  spec_EnvP_bProvDef/1 -> BC/5  "testSig_EnvP_bProvDef"
  spec_EnvP_bPhysRngFinalDef/1 -> BC/6  "testSig_EnvP_bPhysRngFinalDef"
  spec_EnvP_bPhysRngProvDef/1 -> BC/7  "testSig_EnvP_bPhysRngProvDef"
  spec_EnvP_bSRCMaxDeb_DSM/1 -> BC/8  "testSig_EnvP_bSRCMaxDeb_DSM"
  spec_EnvP_bSRCMinDeb_DSM/1 -> BC/9  "testSig_EnvP_bSRCMinDeb_DSM"
  spec_EnvP_bPhysRngHiDeb_DSM/1 -> BC/10  "testSig_EnvP_bPhysRngHiDeb_DSM"
  spec_EnvP_bPhysRngLoDeb_DSM/1 -> BC/11  "testSig_EnvP_bPhysRngLoDeb_DSM"

== system TST_EnvP_DD/simulationInput/testSignals_R003 ==
  BC : BusCreator  Inputs=11
  spec_DSM_bEnvPSS : FromWorkspace  VariableName=testSig_DSM_bEnvPSS  Interpolate=off  OutputAfterFinalValue=Holding final value
  spec_EnvP_bFinalDef : FromWorkspace  VariableName=testSig_EnvP_bFinalDef  Interpolate=off  OutputAfterFinalValue=Holding final value
  spec_EnvP_bPhysRngFinalDef : FromWorkspace  VariableName=testSig_EnvP_bPhysRngFinalDef  Interpolate=off  OutputAfterFinalValue=Holding final value
  spec_EnvP_bPhysRngHiDeb_DSM : FromWorkspace  VariableName=testSig_EnvP_bPhysRngHiDeb_DSM  Interpolate=off  OutputAfterFinalValue=Holding final value
  spec_EnvP_bPhysRngLoDeb_DSM : FromWorkspace  VariableName=testSig_EnvP_bPhysRngLoDeb_DSM  Interpolate=off  OutputAfterFinalValue=Holding final value
  spec_EnvP_bPhysRngProvDef : FromWorkspace  VariableName=testSig_EnvP_bPhysRngProvDef  Interpolate=off  OutputAfterFinalValue=Holding final value
  spec_EnvP_bProvDef : FromWorkspace  VariableName=testSig_EnvP_bProvDef  Interpolate=off  OutputAfterFinalValue=Holding final value
  spec_EnvP_bSRCMaxDeb_DSM : FromWorkspace  VariableName=testSig_EnvP_bSRCMaxDeb_DSM  Interpolate=off  OutputAfterFinalValue=Holding final value
  spec_EnvP_bSRCMinDeb_DSM : FromWorkspace  VariableName=testSig_EnvP_bSRCMinDeb_DSM  Interpolate=off  OutputAfterFinalValue=Holding final value
  spec_EnvP_pSens : FromWorkspace  VariableName=testSig_EnvP_pSens  Interpolate=off  OutputAfterFinalValue=Holding final value
  spec_EnvP_uRaw : FromWorkspace  VariableName=testSig_EnvP_uRaw  Interpolate=off  OutputAfterFinalValue=Holding final value
  testSignals : Outport
  wires:
  BC/1 -> testSignals/1
  spec_EnvP_uRaw/1 -> BC/1  "testSig_EnvP_uRaw"
  spec_DSM_bEnvPSS/1 -> BC/2  "testSig_DSM_bEnvPSS"
  spec_EnvP_pSens/1 -> BC/3  "testSig_EnvP_pSens"
  spec_EnvP_bFinalDef/1 -> BC/4  "testSig_EnvP_bFinalDef"
  spec_EnvP_bProvDef/1 -> BC/5  "testSig_EnvP_bProvDef"
  spec_EnvP_bPhysRngFinalDef/1 -> BC/6  "testSig_EnvP_bPhysRngFinalDef"
  spec_EnvP_bPhysRngProvDef/1 -> BC/7  "testSig_EnvP_bPhysRngProvDef"
  spec_EnvP_bSRCMaxDeb_DSM/1 -> BC/8  "testSig_EnvP_bSRCMaxDeb_DSM"
  spec_EnvP_bSRCMinDeb_DSM/1 -> BC/9  "testSig_EnvP_bSRCMinDeb_DSM"
  spec_EnvP_bPhysRngHiDeb_DSM/1 -> BC/10  "testSig_EnvP_bPhysRngHiDeb_DSM"
  spec_EnvP_bPhysRngLoDeb_DSM/1 -> BC/11  "testSig_EnvP_bPhysRngLoDeb_DSM"

== system TST_EnvP_DD/simulationInput/testSignals_R004 ==
  BC : BusCreator  Inputs=11
  spec_DSM_bEnvPSS : FromWorkspace  VariableName=testSig_DSM_bEnvPSS  Interpolate=off  OutputAfterFinalValue=Holding final value
  spec_EnvP_bFinalDef : FromWorkspace  VariableName=testSig_EnvP_bFinalDef  Interpolate=off  OutputAfterFinalValue=Holding final value
  spec_EnvP_bPhysRngFinalDef : FromWorkspace  VariableName=testSig_EnvP_bPhysRngFinalDef  Interpolate=off  OutputAfterFinalValue=Holding final value
  spec_EnvP_bPhysRngHiDeb_DSM : FromWorkspace  VariableName=testSig_EnvP_bPhysRngHiDeb_DSM  Interpolate=off  OutputAfterFinalValue=Holding final value
  spec_EnvP_bPhysRngLoDeb_DSM : FromWorkspace  VariableName=testSig_EnvP_bPhysRngLoDeb_DSM  Interpolate=off  OutputAfterFinalValue=Holding final value
  spec_EnvP_bPhysRngProvDef : FromWorkspace  VariableName=testSig_EnvP_bPhysRngProvDef  Interpolate=off  OutputAfterFinalValue=Holding final value
  spec_EnvP_bProvDef : FromWorkspace  VariableName=testSig_EnvP_bProvDef  Interpolate=off  OutputAfterFinalValue=Holding final value
  spec_EnvP_bSRCMaxDeb_DSM : FromWorkspace  VariableName=testSig_EnvP_bSRCMaxDeb_DSM  Interpolate=off  OutputAfterFinalValue=Holding final value
  spec_EnvP_bSRCMinDeb_DSM : FromWorkspace  VariableName=testSig_EnvP_bSRCMinDeb_DSM  Interpolate=off  OutputAfterFinalValue=Holding final value
  spec_EnvP_pSens : FromWorkspace  VariableName=testSig_EnvP_pSens  Interpolate=off  OutputAfterFinalValue=Holding final value
  spec_EnvP_uRaw : FromWorkspace  VariableName=testSig_EnvP_uRaw  Interpolate=off  OutputAfterFinalValue=Holding final value
  testSignals : Outport
  wires:
  BC/1 -> testSignals/1
  spec_EnvP_uRaw/1 -> BC/1  "testSig_EnvP_uRaw"
  spec_DSM_bEnvPSS/1 -> BC/2  "testSig_DSM_bEnvPSS"
  spec_EnvP_pSens/1 -> BC/3  "testSig_EnvP_pSens"
  spec_EnvP_bFinalDef/1 -> BC/4  "testSig_EnvP_bFinalDef"
  spec_EnvP_bProvDef/1 -> BC/5  "testSig_EnvP_bProvDef"
  spec_EnvP_bPhysRngFinalDef/1 -> BC/6  "testSig_EnvP_bPhysRngFinalDef"
  spec_EnvP_bPhysRngProvDef/1 -> BC/7  "testSig_EnvP_bPhysRngProvDef"
  spec_EnvP_bSRCMaxDeb_DSM/1 -> BC/8  "testSig_EnvP_bSRCMaxDeb_DSM"
  spec_EnvP_bSRCMinDeb_DSM/1 -> BC/9  "testSig_EnvP_bSRCMinDeb_DSM"
  spec_EnvP_bPhysRngHiDeb_DSM/1 -> BC/10  "testSig_EnvP_bPhysRngHiDeb_DSM"
  spec_EnvP_bPhysRngLoDeb_DSM/1 -> BC/11  "testSig_EnvP_bPhysRngLoDeb_DSM"

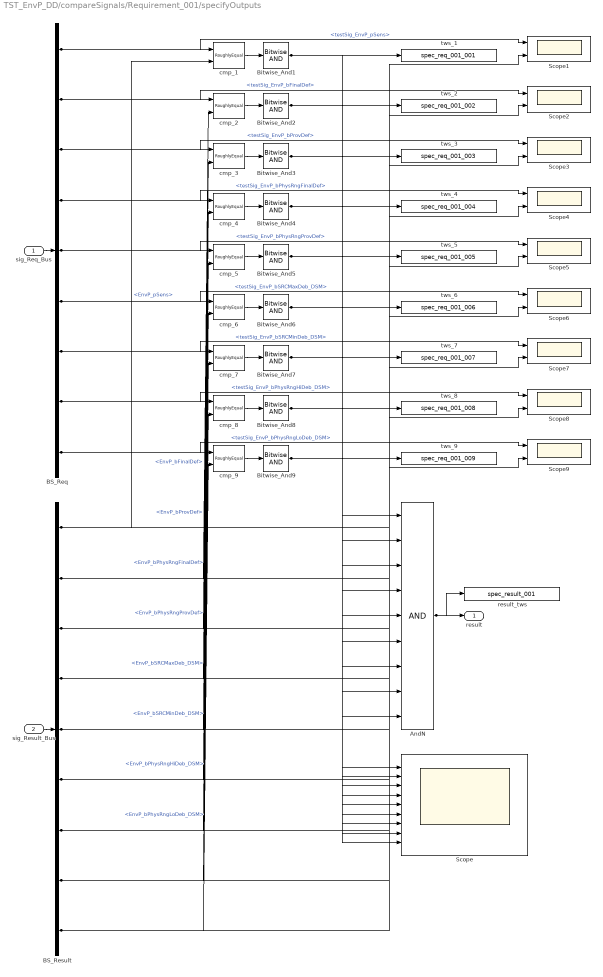
== system TST_EnvP_DD/compareSignals/Requirement_001/specifyOutputs ==
  sig_Req_Bus : Inport
  sig_Result_Bus : Inport  Port=2
  AndN : Logic  Inputs=9
  BS_Req : BusSelector  OutputSignals=testSig_EnvP_pSens,testSig_EnvP_bFinalDef,testSig_EnvP_bProvDef,testSig_EnvP_bPhysRngFinalDef,testSig_EnvP_bPhysRngProvDef,testSig_EnvP_bSRCMaxDeb_DSM,testSig_EnvP_bSRCMinDeb_DSM,testSig_EnvP_bPhysRngHiDeb_DSM,testSig_EnvP_bPhysRngLoDeb_DSM
  BS_Result : BusSelector  OutputSignals=EnvP_pSens,EnvP_bFinalDef,EnvP_bProvDef,EnvP_bPhysRngFinalDef,EnvP_bPhysRngProvDef,EnvP_bSRCMaxDeb_DSM,EnvP_bSRCMinDeb_DSM,EnvP_bPhysRngHiDeb_DSM,EnvP_bPhysRngLoDeb_DSM
  Bitwise_And{1..9} (9 alike) : simulink/Logic and Bit Operations/Bitwise Operator  logicop=AND  UseBitMask=off  BitMask=bin2dec('11011001')  BitMaskRealWorld=Stored Integer
  Scope : Scope  NumInputPorts=9
  Scope{1..9} (9 alike) : Scope  NumInputPorts=2
  cmp_{1..9} (9 alike) : UnitTest_Lib/RoughlyEqual  slope=0.1
  result_tws : ToWorkspace  VariableName=spec_result_001
  tws_1 : ToWorkspace  VariableName=spec_req_001_001
  tws_2 : ToWorkspace  VariableName=spec_req_001_002
  tws_3 : ToWorkspace  VariableName=spec_req_001_003
  tws_4 : ToWorkspace  VariableName=spec_req_001_004
  tws_5 : ToWorkspace  VariableName=spec_req_001_005
  tws_6 : ToWorkspace  VariableName=spec_req_001_006
  tws_7 : ToWorkspace  VariableName=spec_req_001_007
  tws_8 : ToWorkspace  VariableName=spec_req_001_008
  tws_9 : ToWorkspace  VariableName=spec_req_001_009
  result : Outport
  wires:
  sig_Req_Bus/1 -> BS_Req/1
  sig_Result_Bus/1 -> BS_Result/1
  AndN/1 -> result/1, result_tws/1
  BS_Req/1 -> cmp_1/1, Scope1/1  "<testSig_EnvP_pSens>"
  BS_Result/1 -> cmp_1/2, Scope1/2  "<EnvP_pSens>"
  cmp_1/1 -> Bitwise_And1/1
  Bitwise_And1/1 -> tws_1/1, AndN/1, Scope/1
  BS_Req/2 -> cmp_2/1, Scope2/1  "<testSig_EnvP_bFinalDef>"
  BS_Result/2 -> cmp_2/2, Scope2/2  "<EnvP_bFinalDef>"
  cmp_2/1 -> Bitwise_And2/1
  Bitwise_And2/1 -> tws_2/1, AndN/2, Scope/2
  BS_Req/3 -> cmp_3/1, Scope3/1  "<testSig_EnvP_bProvDef>"
  BS_Result/3 -> cmp_3/2, Scope3/2  "<EnvP_bProvDef>"
  cmp_3/1 -> Bitwise_And3/1
  Bitwise_And3/1 -> tws_3/1, AndN/3, Scope/3
  BS_Req/4 -> cmp_4/1, Scope4/1  "<testSig_EnvP_bPhysRngFinalDef>"
  BS_Result/4 -> cmp_4/2, Scope4/2  "<EnvP_bPhysRngFinalDef>"
  cmp_4/1 -> Bitwise_And4/1
  Bitwise_And4/1 -> tws_4/1, AndN/4, Scope/4
  BS_Req/5 -> cmp_5/1, Scope5/1  "<testSig_EnvP_bPhysRngProvDef>"
  BS_Result/5 -> cmp_5/2, Scope5/2  "<EnvP_bPhysRngProvDef>"
  cmp_5/1 -> Bitwise_And5/1
  Bitwise_And5/1 -> tws_5/1, AndN/5, Scope/5
  BS_Req/6 -> cmp_6/1, Scope6/1  "<testSig_EnvP_bSRCMaxDeb_DSM>"
  BS_Result/6 -> cmp_6/2, Scope6/2  "<EnvP_bSRCMaxDeb_DSM>"
  cmp_6/1 -> Bitwise_And6/1
  Bitwise_And6/1 -> tws_6/1, AndN/6, Scope/6
  BS_Req/7 -> cmp_7/1, Scope7/1  "<testSig_EnvP_bSRCMinDeb_DSM>"
  BS_Result/7 -> cmp_7/2, Scope7/2  "<EnvP_bSRCMinDeb_DSM>"
  cmp_7/1 -> Bitwise_And7/1
  Bitwise_And7/1 -> tws_7/1, AndN/7, Scope/7
  BS_Req/8 -> cmp_8/1, Scope8/1  "<testSig_EnvP_bPhysRngHiDeb_DSM>"
  BS_Result/8 -> cmp_8/2, Scope8/2  "<EnvP_bPhysRngHiDeb_DSM>"
  cmp_8/1 -> Bitwise_And8/1
  Bitwise_And8/1 -> tws_8/1, AndN/8, Scope/8
  BS_Req/9 -> cmp_9/1, Scope9/1  "<testSig_EnvP_bPhysRngLoDeb_DSM>"
  BS_Result/9 -> cmp_9/2, Scope9/2  "<EnvP_bPhysRngLoDeb_DSM>"
  cmp_9/1 -> Bitwise_And9/1
  Bitwise_And9/1 -> tws_9/1, AndN/9, Scope/9

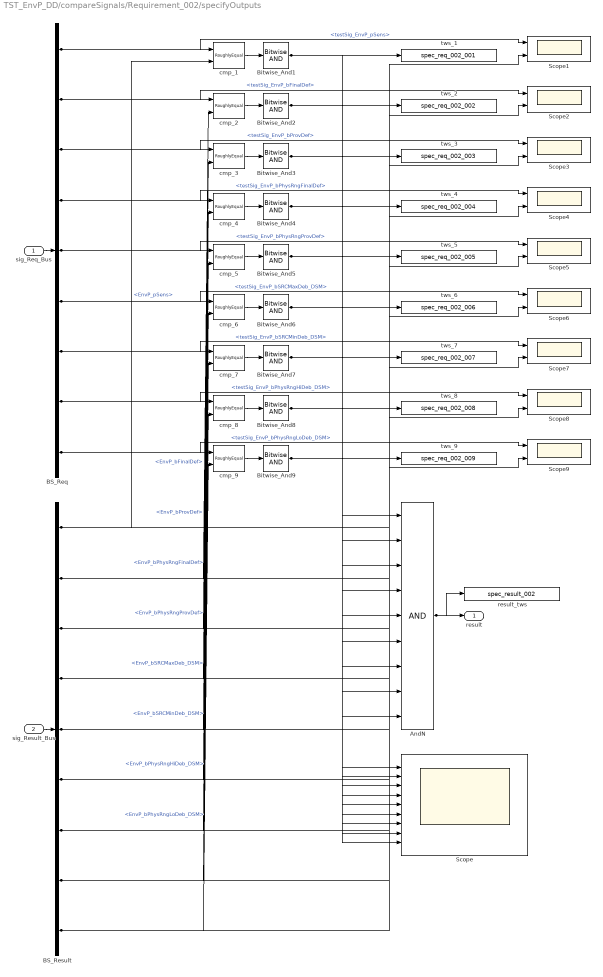
== system TST_EnvP_DD/compareSignals/Requirement_002/specifyOutputs ==
  sig_Req_Bus : Inport
  sig_Result_Bus : Inport  Port=2
  AndN : Logic  Inputs=9
  BS_Req : BusSelector  OutputSignals=testSig_EnvP_pSens,testSig_EnvP_bFinalDef,testSig_EnvP_bProvDef,testSig_EnvP_bPhysRngFinalDef,testSig_EnvP_bPhysRngProvDef,testSig_EnvP_bSRCMaxDeb_DSM,testSig_EnvP_bSRCMinDeb_DSM,testSig_EnvP_bPhysRngHiDeb_DSM,testSig_EnvP_bPhysRngLoDeb_DSM
  BS_Result : BusSelector  OutputSignals=EnvP_pSens,EnvP_bFinalDef,EnvP_bProvDef,EnvP_bPhysRngFinalDef,EnvP_bPhysRngProvDef,EnvP_bSRCMaxDeb_DSM,EnvP_bSRCMinDeb_DSM,EnvP_bPhysRngHiDeb_DSM,EnvP_bPhysRngLoDeb_DSM
  Bitwise_And{1..9} (9 alike) : simulink/Logic and Bit Operations/Bitwise Operator  logicop=AND  UseBitMask=off  BitMask=bin2dec('11011001')  BitMaskRealWorld=Stored Integer
  Scope : Scope  NumInputPorts=9
  Scope{1..9} (9 alike) : Scope  NumInputPorts=2
  cmp_{1..9} (9 alike) : UnitTest_Lib/RoughlyEqual  slope=0.1
  result_tws : ToWorkspace  VariableName=spec_result_002
  tws_1 : ToWorkspace  VariableName=spec_req_002_001
  tws_2 : ToWorkspace  VariableName=spec_req_002_002
  tws_3 : ToWorkspace  VariableName=spec_req_002_003
  tws_4 : ToWorkspace  VariableName=spec_req_002_004
  tws_5 : ToWorkspace  VariableName=spec_req_002_005
  tws_6 : ToWorkspace  VariableName=spec_req_002_006
  tws_7 : ToWorkspace  VariableName=spec_req_002_007
  tws_8 : ToWorkspace  VariableName=spec_req_002_008
  tws_9 : ToWorkspace  VariableName=spec_req_002_009
  result : Outport
  wires:
  sig_Req_Bus/1 -> BS_Req/1
  sig_Result_Bus/1 -> BS_Result/1
  AndN/1 -> result/1, result_tws/1
  BS_Req/1 -> cmp_1/1, Scope1/1  "<testSig_EnvP_pSens>"
  BS_Result/1 -> cmp_1/2, Scope1/2  "<EnvP_pSens>"
  cmp_1/1 -> Bitwise_And1/1
  Bitwise_And1/1 -> tws_1/1, AndN/1, Scope/1
  BS_Req/2 -> cmp_2/1, Scope2/1  "<testSig_EnvP_bFinalDef>"
  BS_Result/2 -> cmp_2/2, Scope2/2  "<EnvP_bFinalDef>"
  cmp_2/1 -> Bitwise_And2/1
  Bitwise_And2/1 -> tws_2/1, AndN/2, Scope/2
  BS_Req/3 -> cmp_3/1, Scope3/1  "<testSig_EnvP_bProvDef>"
  BS_Result/3 -> cmp_3/2, Scope3/2  "<EnvP_bProvDef>"
  cmp_3/1 -> Bitwise_And3/1
  Bitwise_And3/1 -> tws_3/1, AndN/3, Scope/3
  BS_Req/4 -> cmp_4/1, Scope4/1  "<testSig_EnvP_bPhysRngFinalDef>"
  BS_Result/4 -> cmp_4/2, Scope4/2  "<EnvP_bPhysRngFinalDef>"
  cmp_4/1 -> Bitwise_And4/1
  Bitwise_And4/1 -> tws_4/1, AndN/4, Scope/4
  BS_Req/5 -> cmp_5/1, Scope5/1  "<testSig_EnvP_bPhysRngProvDef>"
  BS_Result/5 -> cmp_5/2, Scope5/2  "<EnvP_bPhysRngProvDef>"
  cmp_5/1 -> Bitwise_And5/1
  Bitwise_And5/1 -> tws_5/1, AndN/5, Scope/5
  BS_Req/6 -> cmp_6/1, Scope6/1  "<testSig_EnvP_bSRCMaxDeb_DSM>"
  BS_Result/6 -> cmp_6/2, Scope6/2  "<EnvP_bSRCMaxDeb_DSM>"
  cmp_6/1 -> Bitwise_And6/1
  Bitwise_And6/1 -> tws_6/1, AndN/6, Scope/6
  BS_Req/7 -> cmp_7/1, Scope7/1  "<testSig_EnvP_bSRCMinDeb_DSM>"
  BS_Result/7 -> cmp_7/2, Scope7/2  "<EnvP_bSRCMinDeb_DSM>"
  cmp_7/1 -> Bitwise_And7/1
  Bitwise_And7/1 -> tws_7/1, AndN/7, Scope/7
  BS_Req/8 -> cmp_8/1, Scope8/1  "<testSig_EnvP_bPhysRngHiDeb_DSM>"
  BS_Result/8 -> cmp_8/2, Scope8/2  "<EnvP_bPhysRngHiDeb_DSM>"
  cmp_8/1 -> Bitwise_And8/1
  Bitwise_And8/1 -> tws_8/1, AndN/8, Scope/8
  BS_Req/9 -> cmp_9/1, Scope9/1  "<testSig_EnvP_bPhysRngLoDeb_DSM>"
  BS_Result/9 -> cmp_9/2, Scope9/2  "<EnvP_bPhysRngLoDeb_DSM>"
  cmp_9/1 -> Bitwise_And9/1
  Bitwise_And9/1 -> tws_9/1, AndN/9, Scope/9

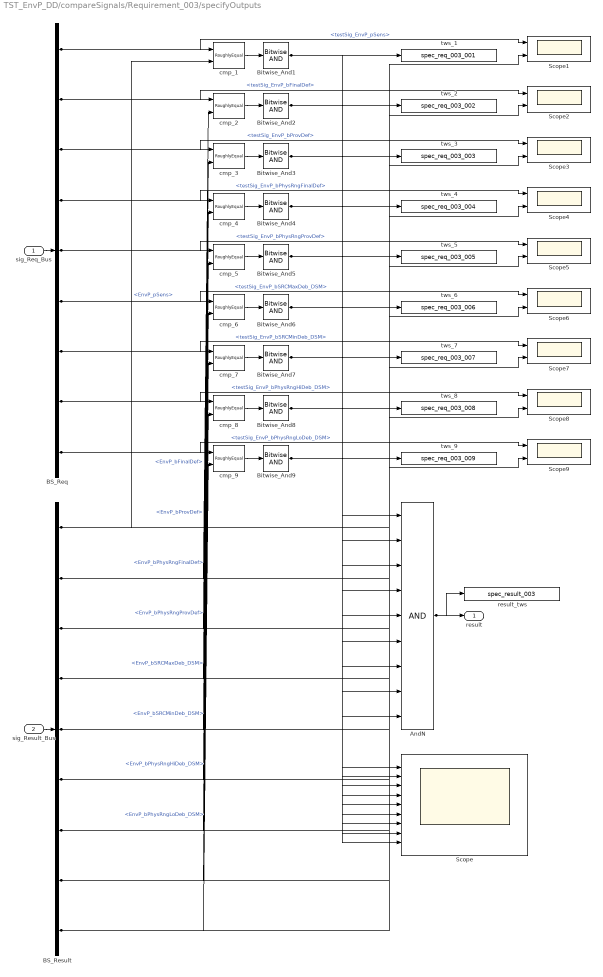
== system TST_EnvP_DD/compareSignals/Requirement_003/specifyOutputs ==
  sig_Req_Bus : Inport
  sig_Result_Bus : Inport  Port=2
  AndN : Logic  Inputs=9
  BS_Req : BusSelector  OutputSignals=testSig_EnvP_pSens,testSig_EnvP_bFinalDef,testSig_EnvP_bProvDef,testSig_EnvP_bPhysRngFinalDef,testSig_EnvP_bPhysRngProvDef,testSig_EnvP_bSRCMaxDeb_DSM,testSig_EnvP_bSRCMinDeb_DSM,testSig_EnvP_bPhysRngHiDeb_DSM,testSig_EnvP_bPhysRngLoDeb_DSM
  BS_Result : BusSelector  OutputSignals=EnvP_pSens,EnvP_bFinalDef,EnvP_bProvDef,EnvP_bPhysRngFinalDef,EnvP_bPhysRngProvDef,EnvP_bSRCMaxDeb_DSM,EnvP_bSRCMinDeb_DSM,EnvP_bPhysRngHiDeb_DSM,EnvP_bPhysRngLoDeb_DSM
  Bitwise_And{1..9} (9 alike) : simulink/Logic and Bit Operations/Bitwise Operator  logicop=AND  UseBitMask=off  BitMask=bin2dec('11011001')  BitMaskRealWorld=Stored Integer
  Scope : Scope  NumInputPorts=9
  Scope{1..9} (9 alike) : Scope  NumInputPorts=2
  cmp_{1..9} (9 alike) : UnitTest_Lib/RoughlyEqual  slope=0.1
  result_tws : ToWorkspace  VariableName=spec_result_003
  tws_1 : ToWorkspace  VariableName=spec_req_003_001
  tws_2 : ToWorkspace  VariableName=spec_req_003_002
  tws_3 : ToWorkspace  VariableName=spec_req_003_003
  tws_4 : ToWorkspace  VariableName=spec_req_003_004
  tws_5 : ToWorkspace  VariableName=spec_req_003_005
  tws_6 : ToWorkspace  VariableName=spec_req_003_006
  tws_7 : ToWorkspace  VariableName=spec_req_003_007
  tws_8 : ToWorkspace  VariableName=spec_req_003_008
  tws_9 : ToWorkspace  VariableName=spec_req_003_009
  result : Outport
  wires:
  sig_Req_Bus/1 -> BS_Req/1
  sig_Result_Bus/1 -> BS_Result/1
  AndN/1 -> result/1, result_tws/1
  BS_Req/1 -> cmp_1/1, Scope1/1  "<testSig_EnvP_pSens>"
  BS_Result/1 -> cmp_1/2, Scope1/2  "<EnvP_pSens>"
  cmp_1/1 -> Bitwise_And1/1
  Bitwise_And1/1 -> tws_1/1, AndN/1, Scope/1
  BS_Req/2 -> cmp_2/1, Scope2/1  "<testSig_EnvP_bFinalDef>"
  BS_Result/2 -> cmp_2/2, Scope2/2  "<EnvP_bFinalDef>"
  cmp_2/1 -> Bitwise_And2/1
  Bitwise_And2/1 -> tws_2/1, AndN/2, Scope/2
  BS_Req/3 -> cmp_3/1, Scope3/1  "<testSig_EnvP_bProvDef>"
  BS_Result/3 -> cmp_3/2, Scope3/2  "<EnvP_bProvDef>"
  cmp_3/1 -> Bitwise_And3/1
  Bitwise_And3/1 -> tws_3/1, AndN/3, Scope/3
  BS_Req/4 -> cmp_4/1, Scope4/1  "<testSig_EnvP_bPhysRngFinalDef>"
  BS_Result/4 -> cmp_4/2, Scope4/2  "<EnvP_bPhysRngFinalDef>"
  cmp_4/1 -> Bitwise_And4/1
  Bitwise_And4/1 -> tws_4/1, AndN/4, Scope/4
  BS_Req/5 -> cmp_5/1, Scope5/1  "<testSig_EnvP_bPhysRngProvDef>"
  BS_Result/5 -> cmp_5/2, Scope5/2  "<EnvP_bPhysRngProvDef>"
  cmp_5/1 -> Bitwise_And5/1
  Bitwise_And5/1 -> tws_5/1, AndN/5, Scope/5
  BS_Req/6 -> cmp_6/1, Scope6/1  "<testSig_EnvP_bSRCMaxDeb_DSM>"
  BS_Result/6 -> cmp_6/2, Scope6/2  "<EnvP_bSRCMaxDeb_DSM>"
  cmp_6/1 -> Bitwise_And6/1
  Bitwise_And6/1 -> tws_6/1, AndN/6, Scope/6
  BS_Req/7 -> cmp_7/1, Scope7/1  "<testSig_EnvP_bSRCMinDeb_DSM>"
  BS_Result/7 -> cmp_7/2, Scope7/2  "<EnvP_bSRCMinDeb_DSM>"
  cmp_7/1 -> Bitwise_And7/1
  Bitwise_And7/1 -> tws_7/1, AndN/7, Scope/7
  BS_Req/8 -> cmp_8/1, Scope8/1  "<testSig_EnvP_bPhysRngHiDeb_DSM>"
  BS_Result/8 -> cmp_8/2, Scope8/2  "<EnvP_bPhysRngHiDeb_DSM>"
  cmp_8/1 -> Bitwise_And8/1
  Bitwise_And8/1 -> tws_8/1, AndN/8, Scope/8
  BS_Req/9 -> cmp_9/1, Scope9/1  "<testSig_EnvP_bPhysRngLoDeb_DSM>"
  BS_Result/9 -> cmp_9/2, Scope9/2  "<EnvP_bPhysRngLoDeb_DSM>"
  cmp_9/1 -> Bitwise_And9/1
  Bitwise_And9/1 -> tws_9/1, AndN/9, Scope/9

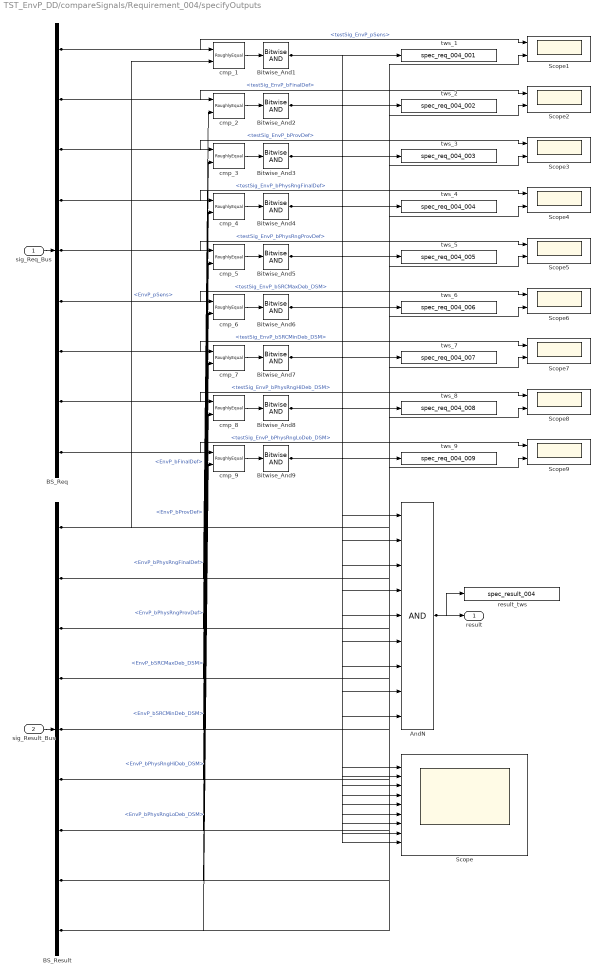
== system TST_EnvP_DD/compareSignals/Requirement_004/specifyOutputs ==
  sig_Req_Bus : Inport
  sig_Result_Bus : Inport  Port=2
  AndN : Logic  Inputs=9
  BS_Req : BusSelector  OutputSignals=testSig_EnvP_pSens,testSig_EnvP_bFinalDef,testSig_EnvP_bProvDef,testSig_EnvP_bPhysRngFinalDef,testSig_EnvP_bPhysRngProvDef,testSig_EnvP_bSRCMaxDeb_DSM,testSig_EnvP_bSRCMinDeb_DSM,testSig_EnvP_bPhysRngHiDeb_DSM,testSig_EnvP_bPhysRngLoDeb_DSM
  BS_Result : BusSelector  OutputSignals=EnvP_pSens,EnvP_bFinalDef,EnvP_bProvDef,EnvP_bPhysRngFinalDef,EnvP_bPhysRngProvDef,EnvP_bSRCMaxDeb_DSM,EnvP_bSRCMinDeb_DSM,EnvP_bPhysRngHiDeb_DSM,EnvP_bPhysRngLoDeb_DSM
  Bitwise_And{1..9} (9 alike) : simulink/Logic and Bit Operations/Bitwise Operator  logicop=AND  UseBitMask=off  BitMask=bin2dec('11011001')  BitMaskRealWorld=Stored Integer
  Scope : Scope  NumInputPorts=9
  Scope{1..9} (9 alike) : Scope  NumInputPorts=2
  cmp_{1..9} (9 alike) : UnitTest_Lib/RoughlyEqual  slope=0.1
  result_tws : ToWorkspace  VariableName=spec_result_004
  tws_1 : ToWorkspace  VariableName=spec_req_004_001
  tws_2 : ToWorkspace  VariableName=spec_req_004_002
  tws_3 : ToWorkspace  VariableName=spec_req_004_003
  tws_4 : ToWorkspace  VariableName=spec_req_004_004
  tws_5 : ToWorkspace  VariableName=spec_req_004_005
  tws_6 : ToWorkspace  VariableName=spec_req_004_006
  tws_7 : ToWorkspace  VariableName=spec_req_004_007
  tws_8 : ToWorkspace  VariableName=spec_req_004_008
  tws_9 : ToWorkspace  VariableName=spec_req_004_009
  result : Outport
  wires:
  sig_Req_Bus/1 -> BS_Req/1
  sig_Result_Bus/1 -> BS_Result/1
  AndN/1 -> result/1, result_tws/1
  BS_Req/1 -> cmp_1/1, Scope1/1  "<testSig_EnvP_pSens>"
  BS_Result/1 -> cmp_1/2, Scope1/2  "<EnvP_pSens>"
  cmp_1/1 -> Bitwise_And1/1
  Bitwise_And1/1 -> tws_1/1, AndN/1, Scope/1
  BS_Req/2 -> cmp_2/1, Scope2/1  "<testSig_EnvP_bFinalDef>"
  BS_Result/2 -> cmp_2/2, Scope2/2  "<EnvP_bFinalDef>"
  cmp_2/1 -> Bitwise_And2/1
  Bitwise_And2/1 -> tws_2/1, AndN/2, Scope/2
  BS_Req/3 -> cmp_3/1, Scope3/1  "<testSig_EnvP_bProvDef>"
  BS_Result/3 -> cmp_3/2, Scope3/2  "<EnvP_bProvDef>"
  cmp_3/1 -> Bitwise_And3/1
  Bitwise_And3/1 -> tws_3/1, AndN/3, Scope/3
  BS_Req/4 -> cmp_4/1, Scope4/1  "<testSig_EnvP_bPhysRngFinalDef>"
  BS_Result/4 -> cmp_4/2, Scope4/2  "<EnvP_bPhysRngFinalDef>"
  cmp_4/1 -> Bitwise_And4/1
  Bitwise_And4/1 -> tws_4/1, AndN/4, Scope/4
  BS_Req/5 -> cmp_5/1, Scope5/1  "<testSig_EnvP_bPhysRngProvDef>"
  BS_Result/5 -> cmp_5/2, Scope5/2  "<EnvP_bPhysRngProvDef>"
  cmp_5/1 -> Bitwise_And5/1
  Bitwise_And5/1 -> tws_5/1, AndN/5, Scope/5
  BS_Req/6 -> cmp_6/1, Scope6/1  "<testSig_EnvP_bSRCMaxDeb_DSM>"
  BS_Result/6 -> cmp_6/2, Scope6/2  "<EnvP_bSRCMaxDeb_DSM>"
  cmp_6/1 -> Bitwise_And6/1
  Bitwise_And6/1 -> tws_6/1, AndN/6, Scope/6
  BS_Req/7 -> cmp_7/1, Scope7/1  "<testSig_EnvP_bSRCMinDeb_DSM>"
  BS_Result/7 -> cmp_7/2, Scope7/2  "<EnvP_bSRCMinDeb_DSM>"
  cmp_7/1 -> Bitwise_And7/1
  Bitwise_And7/1 -> tws_7/1, AndN/7, Scope/7
  BS_Req/8 -> cmp_8/1, Scope8/1  "<testSig_EnvP_bPhysRngHiDeb_DSM>"
  BS_Result/8 -> cmp_8/2, Scope8/2  "<EnvP_bPhysRngHiDeb_DSM>"
  cmp_8/1 -> Bitwise_And8/1
  Bitwise_And8/1 -> tws_8/1, AndN/8, Scope/8
  BS_Req/9 -> cmp_9/1, Scope9/1  "<testSig_EnvP_bPhysRngLoDeb_DSM>"
  BS_Result/9 -> cmp_9/2, Scope9/2  "<EnvP_bPhysRngLoDeb_DSM>"
  cmp_9/1 -> Bitwise_And9/1
  Bitwise_And9/1 -> tws_9/1, AndN/9, Scope/9
